simulink model "observer_kahesh"  (R2018b)
settings: Solver=VariableStepAuto  StartTime=0.0  StopTime=100  RelTol=1e-3  EnableMultiTasking=on
settings Model: Creator=mac  LastModifiedBy=sepehr
settings DataIOCC: LimitDataPoints=on
settings OptimizationCC: LifeSpan=inf
settings DebuggingCC: AllowSymbolicDim=off  SFUnexpectedBacktrackingDiag=warning  SFNoUnconditionalDefaultTransitionDiag=warning  SFExecutionAtInitializationDiag=none
settings ModelReferenceCC: PropagateSignalLabelsOutOfModel=off
settings SFSimCC: SimUseLocalCustomCode=off
settings RTWCC: RTWUseLocalCustomCode=off
settings CodeAppCC: StateflowObjectComments=on
settings GRTTargetCC: TargetLangStandard=C89/C90 (ANSI)
settings ConfigComp: CovMetricSettings=dw  CovHtmlReporting=on  CovSaveCumulativeToWorkspaceVar=on  CovSaveSingleToWorkspaceVar=on  CovExternalEMLEnable=off

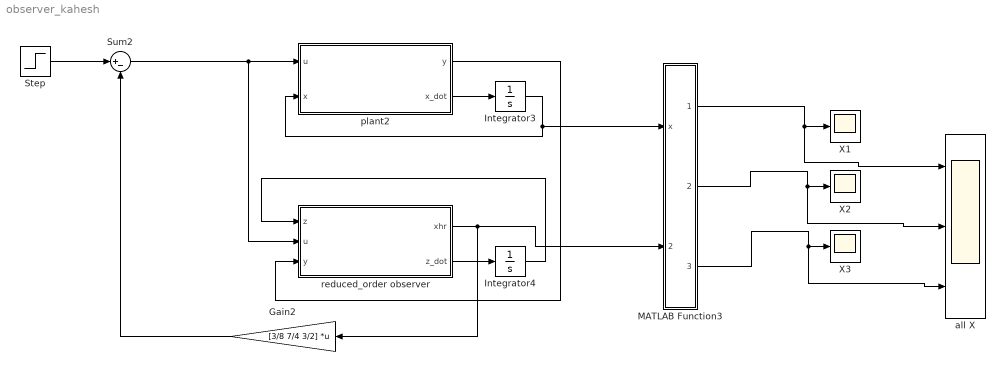
== system observer_kahesh ==
  Gain2 : Gain  Gain=[3/8 7/4 3/2]  Multiplication=Matrix(K*u) (u vector)
  Integrator3 : Integrator  InitialCondition=[0 0 0]
  Integrator4 : Integrator  InitialCondition=-0.5
  MATLAB Function3 : MATLAB Function  TreatAsAtomicUnit=on
  Step : Step  After=100  SampleTime=0
  Sum2 : Sum  Inputs=|+-
  X1 : Scope
  X2 : Scope
  X3 : Scope
  all X : Scope  NumInputPorts=3
  plant2 : MATLAB Function  TreatAsAtomicUnit=on
  reduced_order observer : MATLAB Function  TreatAsAtomicUnit=on
  wires:
  plant2/2(x_dot) -> Integrator3/1
  Integrator3/1 -> plant2/2(x), MATLAB Function3/1(x)
  Gain2/1 -> Sum2/2
  Sum2/1 -> reduced_order observer/2(u), plant2/1(u)
  plant2/1(y) -> reduced_order observer/3(y)
  reduced_order observer/2(z_dot) -> Integrator4/1
  Integrator4/1 -> reduced_order observer/1(z)
  reduced_order observer/1(xhr) -> MATLAB Function3/2(x_hat), Gain2/1
  Step/1 -> Sum2/1
  MATLAB Function3/1(x1) -> all X/1, X1/1
  MATLAB Function3/3(x3) -> all X/3, X3/1
  MATLAB Function3/2(x2) -> all X/2, X2/1

== matlab function observer_kahesh/MATLAB Function3 ==
  data: x input; x_hat input; x1 output; x2 output; x3 output
function [x1,x2,x3] = CP(x,x_hat)

x1=[x(1),x_hat(1)];
x2=[x(2),x_hat(2)];
x3=[x(3),x_hat(3)];

== matlab function observer_kahesh/reduced_order observer ==
  data: xhr output; z input; u input; y input; z_dot output
function [xhr,z_dot]= fcn(z,u,y)

D = -10;
R = -19/3;
T = [-10 -121/3];
F1 = [1 11/3; -1 1; 1 0];
F2 = [1;0;0];


z_dot = D*z+ R*u + T*y;
xhr = F1*y+ F2*z;

== matlab function observer_kahesh/plant2 ==
  data: u input; y output; x input; x_dot output
function [y,x_dot]= fcn(u,x)

A = [1 2 0;
     3 -1 1;
     0 2 0];

B = [2;1;1];
C = [0 0 1; 0 1 1];

x_dot = A*x + B*u;
y = C*x;
